simulink model "buildingModel"  (R2017a)
settings: Solver=VariableStepAuto  StartTime=0.0  StopTime=10.0  RelTol=1e-3
values from neighbouring files (symbols this model uses):
  initial_inputs = [0.126, 0.126, 0.126, 0.126, 0.126, 0.126, 0.126, 0.126]    [AdaptiveInitBuilding.m]
  K = zeros(15,1)    [Successive_Linearizer_Building.m]
settings Model: Creator=romanoa5  LastModifiedBy=gaobo1

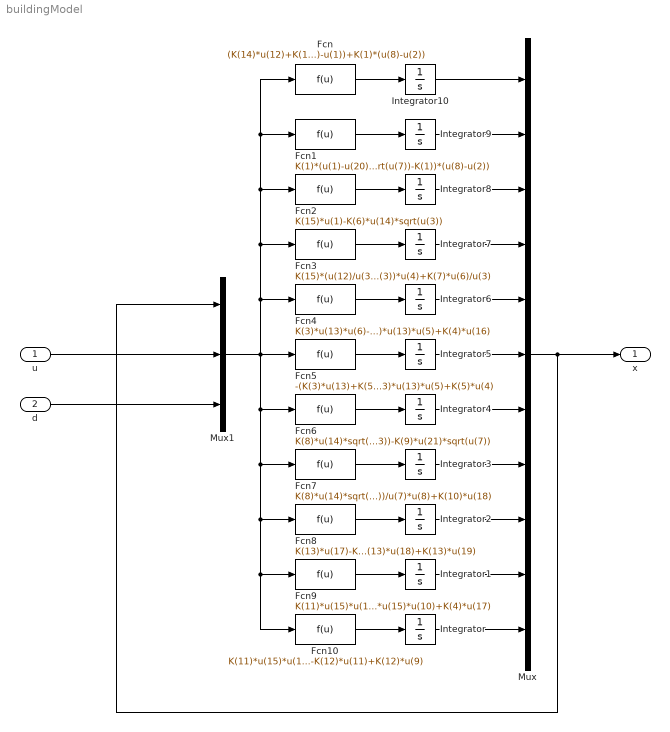
== system buildingModel ==
  u : Inport  OutDataTypeStr=double  PortDimensions=length(initial_inputs)
  d : Inport  Port=2  OutDataTypeStr=double  PortDimensions=2
  Fcn : Fcn  Expr=(K(14)*u(12)+K(1))*(u(20)-u(1))+K(1)*(u(8)-u(2))
  Fcn1 : Fcn  Expr=K(1)*(u(1)-u(20))+(K(2)*u(21)*sqrt(u(7))-K(1))*(u(8)-u(2))
  Fcn10 : Fcn  Expr=K(11)*u(15)*u(1)-K(11)*u(15)*u(11)-K(12)*u(11)+K(12)*u(9)
  Fcn2 : Fcn  Expr=K(15)*u(1)-K(6)*u(14)*sqrt(u(3))
  Fcn3 : Fcn  Expr=K(15)*(u(12)/u(3))*u(1)-(K(15)*(u(12)/u(3))+K(7)/u(3))*u(4)+K(7)*u(6)/u(3)
  Fcn4 : Fcn  Expr=K(3)*u(13)*u(6)-K(3)*u(13)*u(5)+K(4)*u(16)
  Fcn5 : Fcn  Expr=-(K(3)*u(13)+K(5))*u(6)+K(3)*u(13)*u(5)+K(5)*u(4)
  Fcn6 : Fcn  Expr=K(8)*u(14)*sqrt(u(3))-K(9)*u(21)*sqrt(u(7))
  Fcn7 : Fcn  Expr=K(8)*u(14)*sqrt((u(3))/u(7)*u(4))-K(8)*u(14)*sqrt(u(3))/u(7)*u(8)+K(10)*u(18)
  Fcn8 : Fcn  Expr=K(13)*u(17)-K(13)*u(18)+K(13)*u(19)
  Fcn9 : Fcn  Expr=K(11)*u(15)*u(11)-K(11)*u(15)*u(10)+K(4)*u(17)
  Integrator{,1..10} (11 alike) : Integrator
  Mux : Mux  Inputs=11
  Mux1 : Mux  Inputs=3
  x : Outport
  wires:
  Mux/1 -> Mux1/1, x/1
  Fcn/1 -> Integrator10/1
  Fcn1/1 -> Integrator9/1
  Fcn2/1 -> Integrator8/1
  Fcn3/1 -> Integrator7/1
  Fcn4/1 -> Integrator6/1
  Fcn5/1 -> Integrator5/1
  Fcn6/1 -> Integrator4/1
  Fcn7/1 -> Integrator3/1
  Fcn8/1 -> Integrator2/1
  Fcn9/1 -> Integrator1/1
  Fcn10/1 -> Integrator/1
  Integrator10/1 -> Mux/1
  Integrator9/1 -> Mux/2
  Integrator8/1 -> Mux/3
  Integrator7/1 -> Mux/4
  Integrator6/1 -> Mux/5
  Integrator5/1 -> Mux/6
  Integrator4/1 -> Mux/7
  Integrator3/1 -> Mux/8
  Integrator2/1 -> Mux/9
  Integrator1/1 -> Mux/10
  Integrator/1 -> Mux/11
  u/1 -> Mux1/2
  d/1 -> Mux1/3
  Mux1/1 -> Fcn3/1, Fcn2/1, Fcn1/1, Fcn/1, Fcn4/1, Fcn5/1, Fcn6/1, Fcn8/1, Fcn10/1, Fcn9/1, Fcn7/1
